simulink model "testControlWithDroneSwarm"  (R2021b)
settings: Solver=ode4  StartTime=0.0  StopTime=inf  FixedStep=sample_time_base  RelTol=1e-3
InitFcn:
  | init_condition();
StopFcn:
  | stop_function();
values from neighbouring files (symbols this model uses):
  flag_alg = params.swarm_algorithm_type    [init_condition.m]
  inertia = inertia'    [init_condition.m]
  kd_att = kd_att'    [init_condition.m]
  kp_att = kp_att'    [init_condition.m]
  lb_pos_pid = lb_pos_pid'    [init_condition.m]
  lb_vel_pid = lb_vel_pid'    [init_condition.m]
  local_ip = '127.0.0.1'    [init_condition.m]
  motor_init_con = states_omeges(14:17,:)    [init_condition.m]
  number = size(position0,2)    [init_condition.m]
  sample_time_base = 0.0025    [init_condition.m]
  sample_time_control = params.sample_time_control_upper    [init_condition.m]
  sim_quad = param_simulink.sim_quad    [init_condition.m]
  target_ip_array = ones(1,number)*1    [init_condition.m]
  ub_pos_pid = ub_pos_pid'    [init_condition.m]
  ub_vel_pid = ub_vel_pid'    [init_condition.m]
  vehicle_int_con = states_omeges(1:13,:)    [init_condition.m]
undefined symbols (not defined in the file or in its folder): a_max_h, a_max_v, cd_filter_pos, cd_filter_vel, cm, ct, euler_max, get_array_slice, gravity, len_arm, map3d_faces, map3d_struct, mass, T_rotor_inverse, thrust_max, v_max_h, v_max_v, yaw_rate_max
libraries: dspindex x8, aerolibanimutils x1
settings Model: Creator=huangjialei  LastModifiedBy=huangjialei

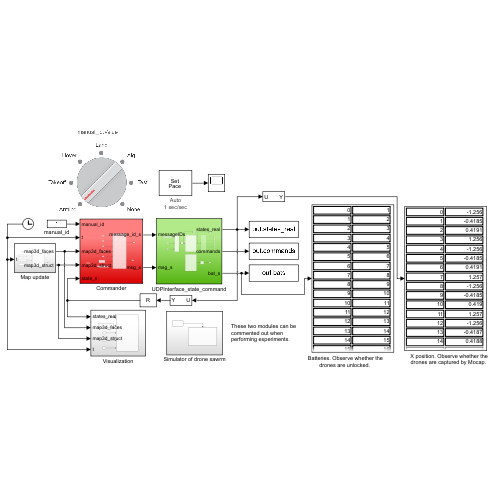
[thumbnail: Simulink's stored preview of the top-level diagram]
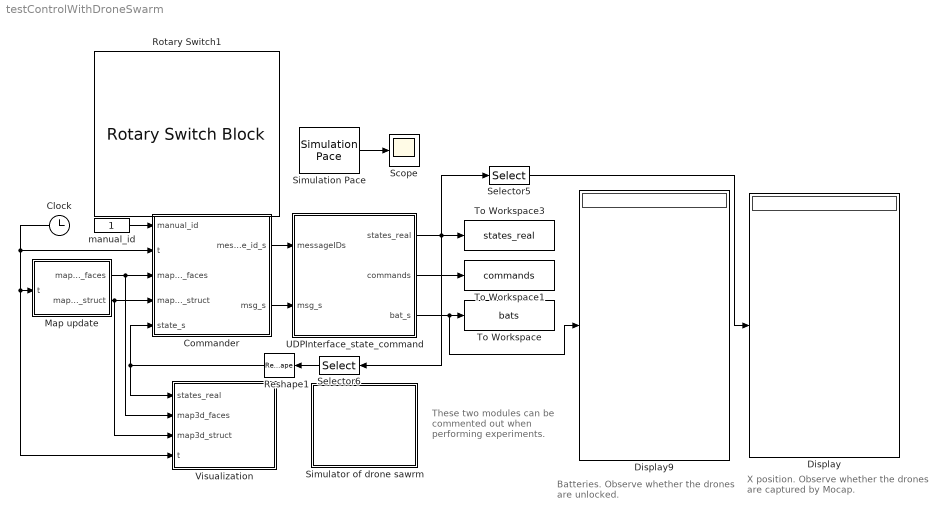
== system testControlWithDroneSwarm ==
  note: These two modules can be commented out when performing experiments.
  note: Batteries. Observe whether the drones are unlocked.
  note: X position. Observe whether the drones are captured by Mocap.
  Clock : Clock
  Commander : Subsystem
  Display : Display
  Display9 : Display
  Map update : Subsystem
  Reshape1 : Reshape  OutputDimensionality=Customize  OutputDimensions=[12,number]
  Rotary Switch1 : RotarySwitchBlock
      settings: Values={{'Arming', 'Takeoff', 'Hover', 'Land', 'Alg', 'Test', 'None'}, [1 2 3 4 5 6 1111]}
  Scope : Scope
  Selector5 : Selector  InputPortWidth=17*number  IndexOptions=Index vector (dialog)  Indices=get_array_slice([1,6], number, 17)  OutputSizes=1
  Selector6 : Selector  InputPortWidth=17*number  IndexOptions=Index vector (dialog)  Indices=get_array_slice(6:17, number, 17)  OutputSizes=1
  Simulation Pace : aerolibanimutils/Simulation Pace  SimulationPace=1  SleepMode=Auto  OutputPaceError=on  SampleTime=sample_time_control
  Simulator of drone sawrm : Subsystem
  To Workspace : ToWorkspace  VariableName=bats  SaveFormat=Timeseries  SampleTime=-1
  To Workspace1 : ToWorkspace  VariableName=commands  SaveFormat=Timeseries  SampleTime=-1
  To Workspace3 : ToWorkspace  VariableName=states_real  SaveFormat=Timeseries  SampleTime=-1
  UDPInterface_state_command : Subsystem
  Visualization : Subsystem
  manual_id : Constant
  wires:
  UDPInterface_state_command/1(states_real) -> Selector6/1, To Workspace3/1, Selector5/1
  Commander/2(msg_s) -> UDPInterface_state_command/2(msg_s)
  UDPInterface_state_command/2(commands) -> To Workspace1/1
  Commander/1(message_id_s) -> UDPInterface_state_command/1(messageIDs)
  UDPInterface_state_command/3(bat_s) -> Display9/1, To Workspace/1
  Selector5/1 -> Display/1
  manual_id/1 -> Commander/1(manual_id)
  Selector6/1 -> Reshape1/1
  Reshape1/1 -> Commander/5(state_s), Visualization/1(states_real)
  Simulation Pace/1 -> Scope/1
  Map update/1(map3d_faces) -> Visualization/2(map3d_faces), Commander/3(map3d_faces)
  Map update/2(map3d_struct) -> Visualization/3(map3d_struct), Commander/4(map3d_struct)
  Clock/1 -> Visualization/4(t), Map update/1(t), Commander/2(t)

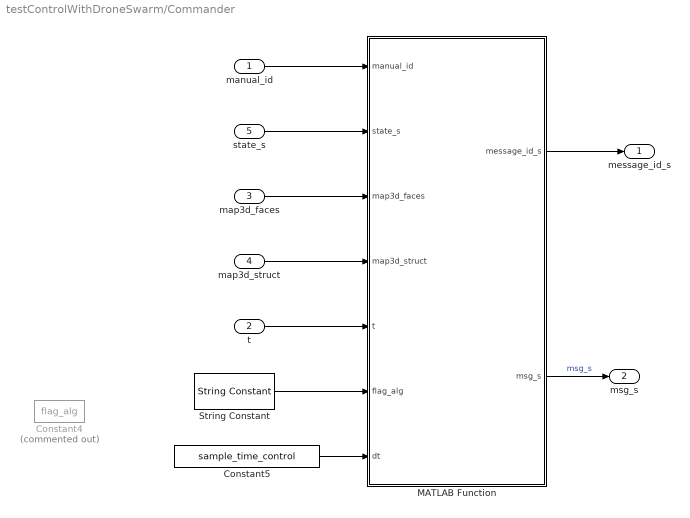
== system testControlWithDroneSwarm/Commander ==
  manual_id : Inport
  t : Inport  Port=2
  map3d_faces : Inport  Port=3
  map3d_struct : Inport  Port=4
  state_s : Inport  Port=5
  Constant4 : Constant  Commented=on  Value=flag_alg
  Constant5 : Constant  Value=sample_time_control
  MATLAB Function : MATLAB Function  TreatAsAtomicUnit=on  SystemSampleTime=sample_time_control
  String Constant : StringConstant  String=flag_alg
  message_id_s : Outport
  msg_s : Outport  Port=2
  wires:
  MATLAB Function/2(msg_s) -> msg_s/1  "msg_s"
  manual_id/1 -> MATLAB Function/1(manual_id)
  t/1 -> MATLAB Function/5(t)
  map3d_faces/1 -> MATLAB Function/3(map3d_faces)
  map3d_struct/1 -> MATLAB Function/4(map3d_struct)
  MATLAB Function/1(message_id_s) -> message_id_s/1
  String Constant/1 -> MATLAB Function/6(flag_alg)
  Constant5/1 -> MATLAB Function/7(dt)
  state_s/1 -> MATLAB Function/2(state_s)

== system testControlWithDroneSwarm/Map update ==
  t : Inport
  Constant : Constant  Value=sample_time_control
  Constant1 : Constant  Value=map3d_faces
  Constant2 : Constant  Value=map3d_struct
  MATLAB Function : MATLAB Function  TreatAsAtomicUnit=on  SystemSampleTime=sample_time_control
  map3d_faces : Outport
  map3d_struct : Outport  Port=2
  wires:
  MATLAB Function/1(map3d_faces) -> map3d_faces/1
  MATLAB Function/2(map3d_struct) -> map3d_struct/1
  t/1 -> MATLAB Function/1(t)
  Constant/1 -> MATLAB Function/2(sample_time_control)
  Constant1/1 -> MATLAB Function/3(map3d_faces_0)
  Constant2/1 -> MATLAB Function/4(map3d_struct_0)

== system testControlWithDroneSwarm/Simulator of drone sawrm ==
  Constant : Constant  Value=sim_quad
  Subsystem : Subsystem
  wires:
  Constant/1 -> Subsystem/Enable

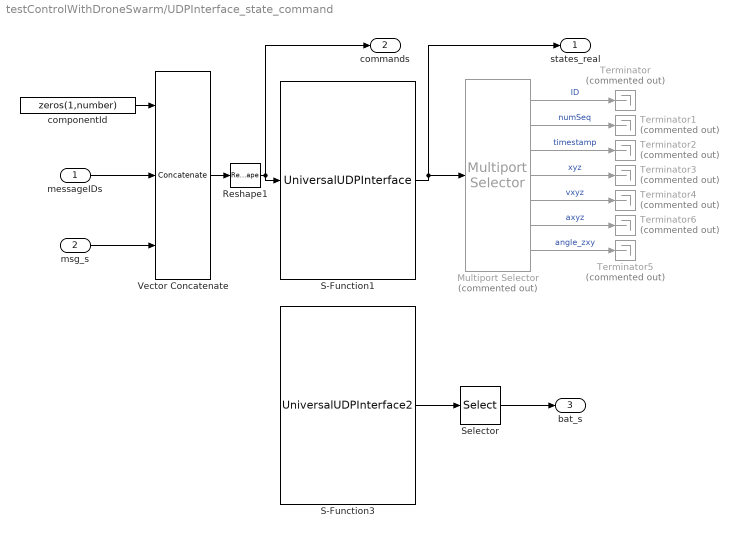
== system testControlWithDroneSwarm/UDPInterface_state_command ==
  messageIDs : Inport
  msg_s : Inport  Port=2
  Multiport Selector : dspindex/Multiport Selector  Commented=on  rowsOrCols=Rows  idxCellArray={1:15:15*number,2:15:15*number,3:15:15*number,repmat(4:6,1,number) + reshape(repmat((0:number-1)*15,3,1),1,3*number), repmat(7:9,1,number) + reshape(repmat((0:number-1)*15,3,1),1,3*number), repmat(10:12,1,number) + reshape(repmat((0:number-1)*15,3,1),1,3*number), repmat(13:15,1,number) + reshape(repmat((0:number-1)*15,3,1),1,3*number)}  idxErrMode=Clip Index
  Reshape1 : Reshape
  S-Function1 : S-Function  FunctionName=UniversalUDPInterface  Parameters=sampleTime,number,portTarget,portLocal,ipTarget,ipLocal,flagSend,flagRecv,inputPortWidth,outputPortWidth  SFunctionDeploymentMode=off  EnableBusSupport=off  mask{number=number, ipLocal=local_ip, ipTarget=target_ip_array, portTarget=21000, portLocal=21000, flagSend=on, flagRecv=on, inputPortWidth=6, outputPortWidth=17, sampleTime=sample_time_control}
      mask prompts: number "Number of vehicles"; ipLocal "Local ip"; ipTarget "Target ip"; portTarget "Start port of target"; portLocal "Start port of local"; flagSend "Enable sender"; flagRecv "Enable receiver"; inputPortWidth "Width of input port"; outputPortWidth "Width of output port"; sampleTime "Sample time"
      mask help:
      | input port: componentId, messageId, msgData[0], msgData[1], ...
      | output port: systemId, numSequence, timeStamp,msgData[0], msgData[1], ...
  S-Function3 : S-Function  FunctionName=UniversalUDPInterface2  Parameters=sampleTime,number,portTarget,portLocal,ipTarget,ipLocal,flagSend,flagRecv,inputPortWidth,outputPortWidth  SFunctionDeploymentMode=off  EnableBusSupport=off  mask{number=number, ipLocal=local_ip, ipTarget=target_ip_array, portTarget=22000, portLocal=20000, flagSend=off, flagRecv=on, inputPortWidth=3, outputPortWidth=6, sampleTime=sample_time_control}
      mask prompts: number "Number of vehicles"; ipLocal "Local ip"; ipTarget "Target ip"; portTarget "Start port of target"; portLocal "Start port of local"; flagSend "Enable sender"; flagRecv "Enable receiver"; inputPortWidth "Width of input port"; outputPortWidth "Width of output port"; sampleTime "Sample time"
      mask help:
      | input port: componentId, messageId, msgData[0], msgData[1], ...
      | output port: systemId, numSequence, timeStamp,msgData[0], msgData[1], ...
  Selector : Selector  InputPortWidth=6*number  IndexOptions=Index vector (dialog)  Indices=get_array_slice([1,6], number, 6)  OutputSizes=1
  Terminator{,1..6} (7 alike) : Terminator  Commented=on
  Vector Concatenate : Concatenate  NumInputs=3  Mode=Multidimensional array
  componentId : Constant  Value=zeros(1,number)  VectorParams1D=off
  states_real : Outport
  commands : Outport  Port=2
  bat_s : Outport  Port=3
  wires:
  Multiport Selector/2 -> Terminator1/1  "numSeq"
  Multiport Selector/5 -> Terminator4/1  "vxyz"
  Vector Concatenate/1 -> Reshape1/1
  Multiport Selector/3 -> Terminator2/1  "timestamp"
  messageIDs/1 -> Vector Concatenate/2
  Reshape1/1 -> S-Function1/1, commands/1
  componentId/1 -> Vector Concatenate/1
  Multiport Selector/4 -> Terminator3/1  "xyz"
  Multiport Selector/1 -> Terminator/1  "ID"
  msg_s/1 -> Vector Concatenate/3
  S-Function3/1 -> Selector/1
  Selector/1 -> bat_s/1
  Multiport Selector/7 -> Terminator5/1  "angle_zxy"
  Multiport Selector/6 -> Terminator6/1  "axyz"
  S-Function1/1 -> states_real/1, Multiport Selector/1

== system testControlWithDroneSwarm/Visualization ==
  states_real : Inport
  map3d_faces : Inport  Port=2
  map3d_struct : Inport  Port=3
  t : Inport  Port=4
  Constant : Constant  Value=sample_time_base
  MATLAB Function : MATLAB Function  TreatAsAtomicUnit=on  SystemSampleTime=sample_time_base
  wires:
  map3d_faces/1 -> MATLAB Function/4(map3d_faces)
  map3d_struct/1 -> MATLAB Function/5(map3d_struct)
  states_real/1 -> MATLAB Function/3(states)
  t/1 -> MATLAB Function/1(t)
  Constant/1 -> MATLAB Function/2(dt)

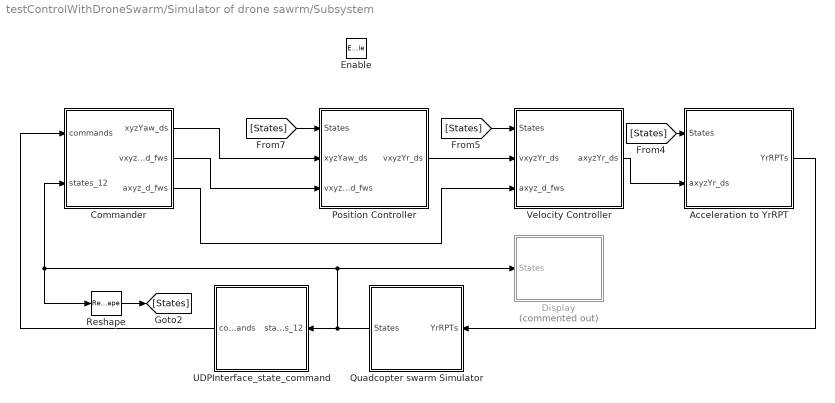
== system testControlWithDroneSwarm/Simulator of drone sawrm/Subsystem ==
  Enable : EnablePort
  Acceleration to YrRPT : Subsystem
  Commander : Subsystem
  Display : Subsystem  Commented=on
  Position Controller : Subsystem
  Quadcopter swarm Simulator : Subsystem
  Reshape : Reshape
  UDPInterface_state_command : Subsystem
  Velocity Controller : Subsystem
  wires:
  Velocity Controller/1(axyzYr_ds) -> Acceleration to YrRPT/2(axyzYr_ds)
  Quadcopter swarm Simulator/1(States) -> UDPInterface_state_command/1(states_12), Commander/2(states_12), Reshape/1, Display/1(States)
  Commander/1(xyzYaw_ds) -> Position Controller/2(xyzYaw_ds)
  Position Controller/1(vxyzYr_ds) -> Velocity Controller/2(vxyzYr_ds)
  UDPInterface_state_command/1(commands) -> Commander/1(commands)
  Reshape/1 -> [States]
  [States] -> Velocity Controller/1(States)
  [States] -> Acceleration to YrRPT/1(States)
  Commander/2(vxyzYr_d_fws) -> Position Controller/3(vxyzYr_d_fws)
  [States] -> Position Controller/1(States)
  Acceleration to YrRPT/1(YrRPTs) -> Quadcopter swarm Simulator/1(YrRPTs)
  Commander/3(axyz_d_fws) -> Velocity Controller/3(axyz_d_fws)

== system testControlWithDroneSwarm/Simulator of drone sawrm/Subsystem/Acceleration to YrRPT ==
  States : Inport
  axyzYr_ds : Inport  Port=2
  Selector : Selector  InputPortWidth=12*number  IndexOptions=Index vector (dialog)  Indices=10:12:12*number  OutputSizes=1
  Subsystem12 : Subsystem
  YrRPTs : Outport
  wires:
  States/1 -> Selector/1
  Selector/1 -> Subsystem12/2(yaws)
  Subsystem12/1(YrRPT) -> YrRPTs/1  "YrRPT"
  axyzYr_ds/1 -> Subsystem12/1(axyzYr_ds)

== system testControlWithDroneSwarm/Simulator of drone sawrm/Subsystem/Commander ==
  commands : Inport
  states_12 : Inport  Port=2
  Clock : Clock
  MATLAB Function : MATLAB Function  TreatAsAtomicUnit=on  SystemSampleTime=sample_time_control
  xyzYaw_ds : Outport
  vxyzYr_d_fws : Outport  Port=2
  axyz_d_fws : Outport  Port=3
  wires:
  Clock/1 -> MATLAB Function/3(t)
  MATLAB Function/2(vxyzYr_ds_fw) -> vxyzYr_d_fws/1
  MATLAB Function/1(xyzYaw_ds) -> xyzYaw_ds/1
  MATLAB Function/3(axyz_ds_fw) -> axyz_d_fws/1
  states_12/1 -> MATLAB Function/2(states)
  commands/1 -> MATLAB Function/1(commands)

== system testControlWithDroneSwarm/Simulator of drone sawrm/Subsystem/Display ==
  States : Inport
  Clock : Clock
  Constant : Constant  Value=len_arm
  MATLAB Function : MATLAB Function  TreatAsAtomicUnit=on  SystemSampleTime=0.1
  wires:
  Constant/1 -> MATLAB Function/2(lenArm)
  Clock/1 -> MATLAB Function/3(t)
  States/1 -> MATLAB Function/1(states)

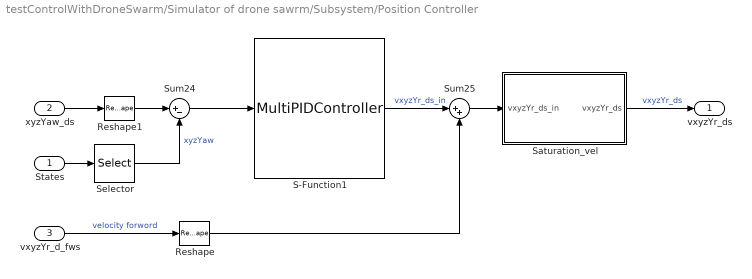
== system testControlWithDroneSwarm/Simulator of drone sawrm/Subsystem/Position Controller ==
  States : Inport
  xyzYaw_ds : Inport  Port=2
  vxyzYr_d_fws : Inport  Port=3
  Reshape : Reshape
  Reshape1 : Reshape
  S-Function1 : S-Function  FunctionName=MultiPIDController  Parameters=sampleTime,number,width,enable_P,enable_I,enable_D,proportion,integral,derivative,c,enable_reset,lb,ub  SFunctionDeploymentMode=off  EnableBusSupport=off  mask{number=number, width=4, enable_P=on, enable_I=on, enable_D=on, proportion=[1,1,1,0], integral=[0,0,0,0], derivative=[0,0,3,0], c=cd_filter_pos, enable_reset=off, lb=lb_pos_pid, ub=ub_pos_pid, sampleTime=sample_time_base}
      mask prompts: number "Number of input port"; width "Width of per input"; enable_P "Enable P"; enable_I "Enable I"; enable_D "Enable D"; c "Coefficient of low-pass filter in derivative part"; enable_reset "Rising edge reset of integral"; lb "Lower boundary of outputs"; ub "Upper boundary of outputs"; sampleTime "Sample time"
      mask Callback enable_P:
      | % disp(get_param(gcbh,'enable_P'))
      | % if strcmp(get_param(gcbh,'enable_P'), 'off')
      | %    disp(get_param(gcbh,'ParameterGroupVar'))
      | %
      | % end
  Saturation_vel : Subsystem
  Selector : Selector  InputPortWidth=12*number  IndexOptions=Index vector (dialog)  Indices=repmat([1,2,3,10],1,number) + reshape(repmat((0:number-1)*12,4,1),1,4*number)  OutputSizes=1
  Sum24 : Sum  Inputs=|+-
  Sum25 : Sum  Inputs=|++
  vxyzYr_ds : Outport
  wires:
  xyzYaw_ds/1 -> Reshape1/1
  States/1 -> Selector/1
  vxyzYr_d_fws/1 -> Reshape/1  "velocity forword"
  Sum24/1 -> S-Function1/1
  Selector/1 -> Sum24/2  "xyzYaw"
  S-Function1/1 -> Sum25/1  "vxyzYr_ds_in"
  Sum25/1 -> Saturation_vel/1(vxyzYr_ds_in)
  Saturation_vel/1(vxyzYr_ds) -> vxyzYr_ds/1  "vxyzYr_ds"
  Reshape/1 -> Sum25/2
  Reshape1/1 -> Sum24/1

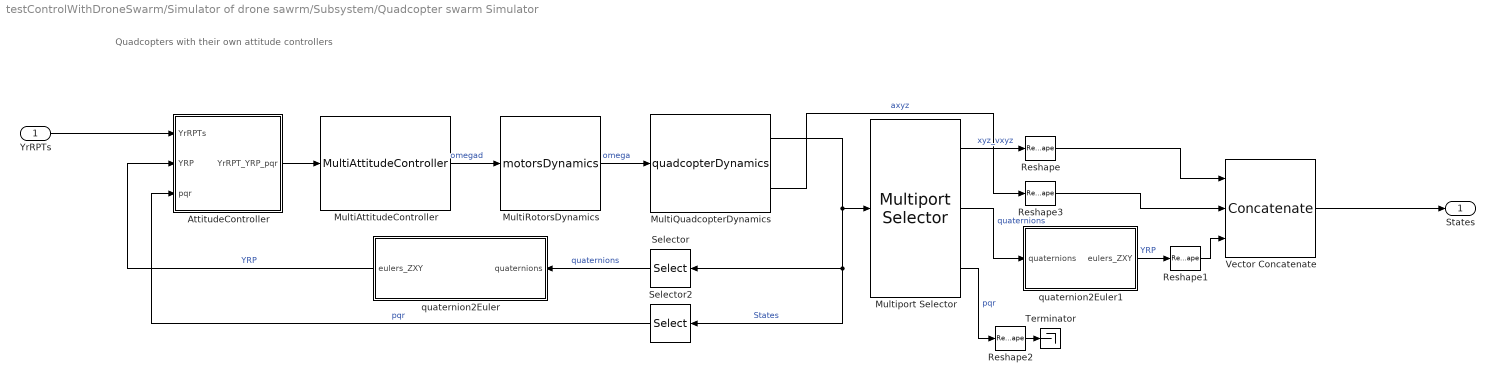
== system testControlWithDroneSwarm/Simulator of drone sawrm/Subsystem/Quadcopter swarm Simulator ==
  note: Quadcopters with their own attitude controllers
  YrRPTs : Inport
  AttitudeController : Subsystem
  MultiAttitudeController : S-Function  FunctionName=MultiAttitudeController  Parameters=number_a,I_a,kp_a,kd_a,arm_length_a,ct_a,cm_a  SFunctionDeploymentMode=off  EnableBusSupport=off  mask{number_a=number+0, I_a=inertia, kp_a=kp_att, kd_a=kd_att, arm_length_a=len_arm, ct_a=ct, cm_a=cm}
      mask prompts: number_a "Number of quadcopters"; I_a "Moment of inertia"; kp_a "Coefficient of proportions"; kd_a "Coefficient of derivatives"; arm_length_a "Length of arm"; ct_a "Thrust coefficient of propeller"; cm_a "Moment coefficient of propeller"
      mask Display:
      | % number = get_param(gcbh,'number_a');
      | % for i = 1:str2num(number)
      | %    port_label('input', i, ['YrRPT_YRP_pqr',num2str(i)]);
      | % end
      | % for i = 1:str2num(number)
      | %    port_label('output', i, ['RPM_d',num2str(i)]);
      | % end
  MultiQuadcopterDynamics : S-Function  FunctionName=quadcopterDynamics  Parameters=number_q,mass_q,I_q,arm_length_q,ct_q,cm_q,conInit_q  SFunctionDeploymentMode=off  EnableBusSupport=off  mask{number_q=number+0, mass_q=mass, I_q=inertia, arm_length_q=len_arm, ct_q=ct, cm_q=cm, conInit_q=vehicle_int_con}
      mask prompts: number_q "Number of quadcopters"; mass_q "Mass"; I_q "Moment of inertia"; arm_length_q "Length of arm"; ct_q "Thrust coefficient of propeller"; cm_q "Moment coefficient of propeller"; conInit_q "Initial condition"
      mask Display:
      | number = get_param(gcbh,'number_q');
      | for i = 1:str2num(number)
      |    port_label('output', i, ['State',num2str(i)]);
      | end
      | for i = 1:str2num(number)
      |    port_label('input', i, ['RPM',num2str(i)]);
      | end
  MultiRotorsDynamics : S-Function  FunctionName=motorsDynamics  Parameters=number_m,K_m,conInit_m  SFunctionDeploymentMode=off  EnableBusSupport=off  mask{number_m=number+0, K_m=T_rotor_inverse, conInit_m=motor_init_con}
      mask prompts: number_m "Number of quadcopters"; K_m "Reciprocal of time constant"; conInit_m "Initial condition"
      mask Display:
      | number = get_param(gcbh,'number_m');
      | for i = 1:str2num(number)
      |    port_label('output', i, ['RPM',num2str(i)]);
      | end
      | for i = 1:str2num(number)
      |    port_label('input', i, ['RPM_d',num2str(i)]);
      | end
  Multiport Selector : dspindex/Multiport Selector  rowsOrCols=Rows  idxCellArray={ repmat(1:6,1,number) + reshape(repmat((0:number-1)*13,6,1),1,6*number),repmat(7:10,1,number) + reshape(repmat((0:number-1)*13,4,1),1,4*number), repmat(11:13,1,number) + reshape(repmat((0:number-1)*13,3,1),1,3*number)}  idxErrMode=Clip Index
  Reshape : Reshape  OutputDimensionality=Customize  OutputDimensions=[6,number]
  Reshape1 : Reshape  OutputDimensionality=Customize  OutputDimensions=[3,number]
  Reshape2 : Reshape  OutputDimensionality=Customize  OutputDimensions=[3,number]
  Reshape3 : Reshape  OutputDimensionality=Customize  OutputDimensions=[3,number]
  Selector : Selector  InputPortWidth=13*number  IndexOptions=Index vector (dialog)  Indices=repmat([7,8,9,10],1,number) + reshape(repmat((0:number-1)*13,4,1),1,4*number)  OutputSizes=1
  Selector2 : Selector  InputPortWidth=13*number  IndexOptions=Index vector (dialog)  Indices=repmat([11,12,13],1,number) + reshape(repmat((0:number-1)*13,3,1),1,3*number)  OutputSizes=1
  Terminator : Terminator
  Vector Concatenate : Concatenate  NumInputs=3  Mode=Multidimensional array
  quaternion2Euler : Subsystem
  quaternion2Euler1 : Subsystem
  States : Outport
  wires:
  YrRPTs/1 -> AttitudeController/1(YrRPTs)
  Selector/1 -> quaternion2Euler/1(quaternions)  "quaternions"
  quaternion2Euler/1(eulers_ZXY) -> AttitudeController/2(YRP)  "YRP"
  Selector2/1 -> AttitudeController/3(pqr)  "pqr"
  MultiAttitudeController/1 -> MultiRotorsDynamics/1  "omegad"
  MultiRotorsDynamics/1 -> MultiQuadcopterDynamics/1  "omega"
  MultiQuadcopterDynamics/1 -> Multiport Selector/1, Selector2/1, Selector/1  "States"
  Multiport Selector/2 -> quaternion2Euler1/1(quaternions)  "quaternions"
  Multiport Selector/1 -> Reshape/1  "xyz_vxyz"
  Reshape/1 -> Vector Concatenate/1
  quaternion2Euler1/1(eulers_ZXY) -> Reshape1/1  "YRP"
  Multiport Selector/3 -> Reshape2/1  "pqr"
  AttitudeController/1(YrRPT_YRP_pqr) -> MultiAttitudeController/1
  Vector Concatenate/1 -> States/1
  Reshape2/1 -> Terminator/1
  Reshape1/1 -> Vector Concatenate/3
  MultiQuadcopterDynamics/2 -> Reshape3/1  "axyz"
  Reshape3/1 -> Vector Concatenate/2

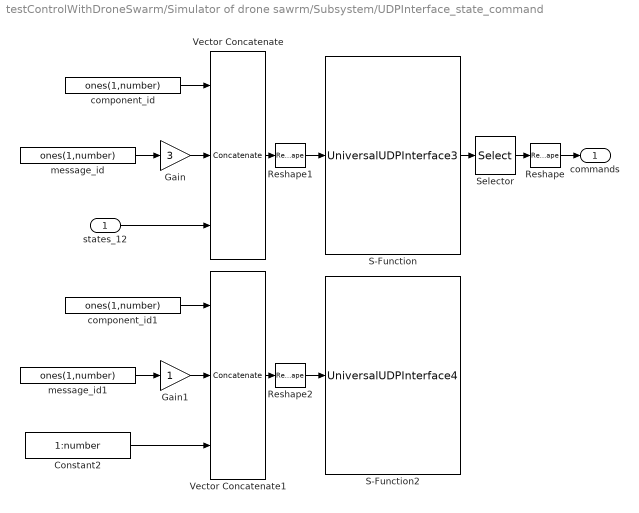
== system testControlWithDroneSwarm/Simulator of drone sawrm/Subsystem/UDPInterface_state_command ==
  states_12 : Inport
  Constant2 : Constant  Value=1:number  VectorParams1D=off
  Gain : Gain  Gain=3
  Gain1 : Gain
  Reshape : Reshape  OutputDimensionality=Customize  OutputDimensions=[6,number]
  Reshape1 : Reshape
  Reshape2 : Reshape
  S-Function : S-Function  FunctionName=UniversalUDPInterface3  Parameters=sampleTime,number,portTarget,portLocal,ipTarget,ipLocal,flagSend,flagRecv,inputPortWidth,outputPortWidth  SFunctionDeploymentMode=off  EnableBusSupport=off  mask{number=number, ipLocal=local_ip, ipTarget=target_ip_array, portTarget=20999, portLocal=21001, flagSend=on, flagRecv=on, inputPortWidth=14, outputPortWidth=9, sampleTime=sample_time_control}
      mask prompts: number "Number of vehicles"; ipLocal "Local ip"; ipTarget "Target ip"; portTarget "Start port of target"; portLocal "Start port of local"; flagSend "Enable sender"; flagRecv "Enable receiver"; inputPortWidth "Width of input port"; outputPortWidth "Width of output port"; sampleTime "Sample time"
      mask help:
      | input port: componentId, messageId, msgData[0], msgData[1], ...
      | output port: systemId, numSequence, timeStamp,msgData[0], msgData[1], ...
  S-Function2 : S-Function  FunctionName=UniversalUDPInterface4  Parameters=sampleTime,number,portTarget,portLocal,ipTarget,ipLocal,flagSend,flagRecv,inputPortWidth,outputPortWidth  SFunctionDeploymentMode=off  EnableBusSupport=off  mask{number=number, ipLocal=local_ip, ipTarget=target_ip_array, portTarget=19999, portLocal=22001, flagSend=on, flagRecv=off, inputPortWidth=3, outputPortWidth=9, sampleTime=sample_time_control}
      mask prompts: number "Number of vehicles"; ipLocal "Local ip"; ipTarget "Target ip"; portTarget "Start port of target"; portLocal "Start port of local"; flagSend "Enable sender"; flagRecv "Enable receiver"; inputPortWidth "Width of input port"; outputPortWidth "Width of output port"; sampleTime "Sample time"
      mask help:
      | input port: componentId, messageId, msgData[0], msgData[1], ...
      | output port: systemId, numSequence, timeStamp,msgData[0], msgData[1], ...
  Selector : Selector  InputPortWidth=9*number  IndexOptions=Index vector (dialog)  Indices=get_array_slice(4:9, number, 9)  OutputSizes=1
  Vector Concatenate : Concatenate  NumInputs=3  Mode=Multidimensional array
  Vector Concatenate1 : Concatenate  NumInputs=3  Mode=Multidimensional array
  component_id : Constant  Value=ones(1,number)  VectorParams1D=off
  component_id1 : Constant  Value=ones(1,number)  VectorParams1D=off
  message_id : Constant  Value=ones(1,number)  VectorParams1D=off
  message_id1 : Constant  Value=ones(1,number)  VectorParams1D=off
  commands : Outport
  wires:
  Vector Concatenate/1 -> Reshape1/1
  Reshape1/1 -> S-Function/1
  component_id/1 -> Vector Concatenate/1
  message_id/1 -> Gain/1
  Gain/1 -> Vector Concatenate/2
  S-Function/1 -> Selector/1
  Gain1/1 -> Vector Concatenate1/2
  message_id1/1 -> Gain1/1
  Constant2/1 -> Vector Concatenate1/3
  component_id1/1 -> Vector Concatenate1/1
  Reshape2/1 -> S-Function2/1
  Vector Concatenate1/1 -> Reshape2/1
  states_12/1 -> Vector Concatenate/3
  Selector/1 -> Reshape/1
  Reshape/1 -> commands/1

== system testControlWithDroneSwarm/Simulator of drone sawrm/Subsystem/Velocity Controller ==
  States : Inport
  vxyzYr_ds : Inport  Port=2
  axyz_d_fws : Inport  Port=3
  Multiport Selector : dspindex/Multiport Selector  rowsOrCols=Rows  idxCellArray={ repmat([1,2,3],1,number) + reshape(repmat((0:number-1)*4,3,1),1,3*number),4:4:4*number}  idxErrMode=Clip Index
  Reshape : Reshape
  S-Function2 : S-Function  FunctionName=MultiPIDController  Parameters=sampleTime,number,width,enable_P,enable_I,enable_D,proportion,integral,derivative,c,enable_reset,lb,ub  SFunctionDeploymentMode=off  EnableBusSupport=off  mask{number=number+0, width=3, enable_P=on, enable_I=on, enable_D=on, proportion=[1.2,1.2,1], integral=[2,2,0.8], derivative=[0.3,0.3,0], c=cd_filter_vel, enable_reset=off, lb=lb_vel_pid, ub=ub_vel_pid, sampleTime=sample_time_base}
      mask prompts: number "Number of input port"; width "Width of per input"; enable_P "Enable P"; enable_I "Enable I"; enable_D "Enable D"; c "Coefficient of low-pass filter in derivative part"; enable_reset "Rising edge reset of integral"; lb "Lower boundary of outputs"; ub "Upper boundary of outputs"; sampleTime "Sample time"
      mask Callback enable_P:
      | % disp(get_param(gcbh,'enable_P'))
      | % if strcmp(get_param(gcbh,'enable_P'), 'off')
      | %    disp(get_param(gcbh,'ParameterGroupVar'))
      | %
      | % end
  Saturation_Acc : Subsystem
  Selector : Selector  InputPortWidth=12*number  IndexOptions=Index vector (dialog)  Indices=repmat([4,5,6],1,number) + reshape(repmat((0:number-1)*12,3,1),1,3*number)  OutputSizes=1
  Sum1 : Sum  Inputs=|++
  Sum2 : Sum  Inputs=|+-
  axyzYr_ds : Outport
  wires:
  States/1 -> Selector/1
  Selector/1 -> Sum2/2  "vxyz"
  Sum2/1 -> S-Function2/1
  Multiport Selector/1 -> Sum2/1  "vxyz_d"
  Multiport Selector/2 -> Saturation_Acc/2(yaw_rates)  "yaw_rate_d"
  vxyzYr_ds/1 -> Multiport Selector/1
  Saturation_Acc/1(axyzYr_ds) -> axyzYr_ds/1  "axyzYs_ds"
  S-Function2/1 -> Sum1/1  "axyzYr_ds_in"
  Sum1/1 -> Saturation_Acc/1(axyz_d_in)
  axyz_d_fws/1 -> Reshape/1
  Reshape/1 -> Sum1/2

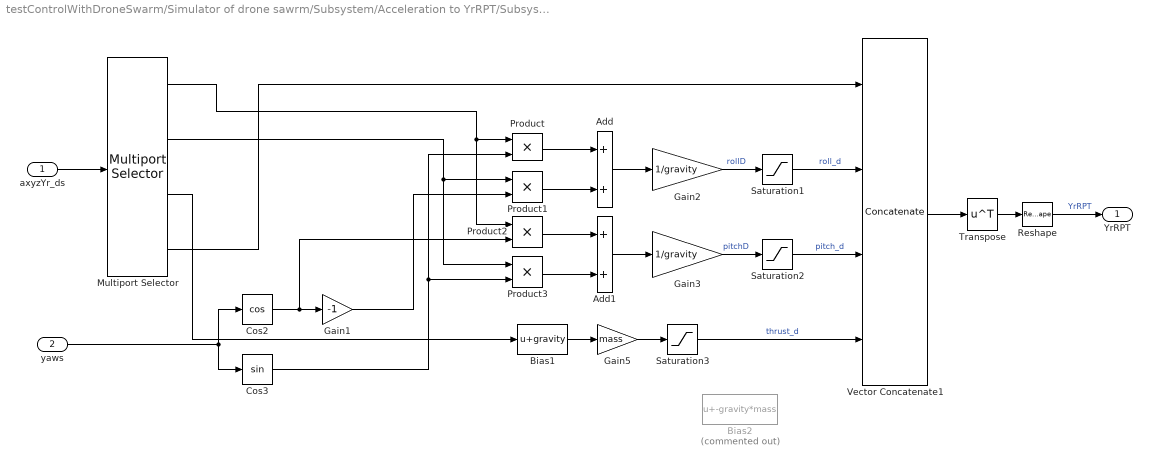
== system testControlWithDroneSwarm/Simulator of drone sawrm/Subsystem/Acceleration to YrRPT/Subsystem12 ==
  axyzYr_ds : Inport
  yaws : Inport  Port=2
  Add : Sum
  Add1 : Sum
  Bias1 : Bias  Bias=gravity
  Bias2 : Bias  Commented=on  Bias=-gravity*mass
  Cos2 : Trigonometry  Operator=cos
  Cos3 : Trigonometry
  Gain1 : Gain  Gain=-1
  Gain2 : Gain  Gain=1/gravity
  Gain3 : Gain  Gain=1/gravity
  Gain5 : Gain  Gain=mass
  Multiport Selector : dspindex/Multiport Selector  rowsOrCols=Rows  idxCellArray={ 1:4:4*number,2:4:4*number, 3:4:4*number,4:4:4*number}  idxErrMode=Clip Index
  Product{,1..3} (4 alike) : Product
  Reshape : Reshape
  Saturation1 : Saturate  UpperLimit=euler_max  LowerLimit=-euler_max
  Saturation2 : Saturate  UpperLimit=euler_max  LowerLimit=-euler_max
  Saturation3 : Saturate  UpperLimit=thrust_max  LowerLimit=0
  Transpose : Math  Operator=transpose  SaturateOnIntegerOverflow=on
  Vector Concatenate1 : Concatenate  NumInputs=4  Mode=Multidimensional array  ConcatenateDimension=2
  YrRPT : Outport
  wires:
  Saturation3/1 -> Vector Concatenate1/4  "thrust_d"
  Saturation2/1 -> Vector Concatenate1/3  "pitch_d"
  Saturation1/1 -> Vector Concatenate1/2  "roll_d"
  Gain5/1 -> Saturation3/1
  Multiport Selector/4 -> Vector Concatenate1/1
  Reshape/1 -> YrRPT/1  "YrRPT"
  Gain2/1 -> Saturation1/1  "rollD"
  Add/1 -> Gain2/1
  Multiport Selector/1 -> Product/1, Product2/1
  Gain1/1 -> Product1/2
  Product/1 -> Add/1
  axyzYr_ds/1 -> Multiport Selector/1
  Product3/1 -> Add1/2
  Cos2/1 -> Gain1/1, Product2/2
  Product1/1 -> Add/2
  Multiport Selector/3 -> Bias1/1
  Gain3/1 -> Saturation2/1  "pitchD"
  Product2/1 -> Add1/1
  Multiport Selector/2 -> Product1/1, Product3/1
  Cos3/1 -> Product3/2, Product/2
  Add1/1 -> Gain3/1
  yaws/1 -> Cos2/1, Cos3/1
  Bias1/1 -> Gain5/1
  Vector Concatenate1/1 -> Transpose/1
  Transpose/1 -> Reshape/1

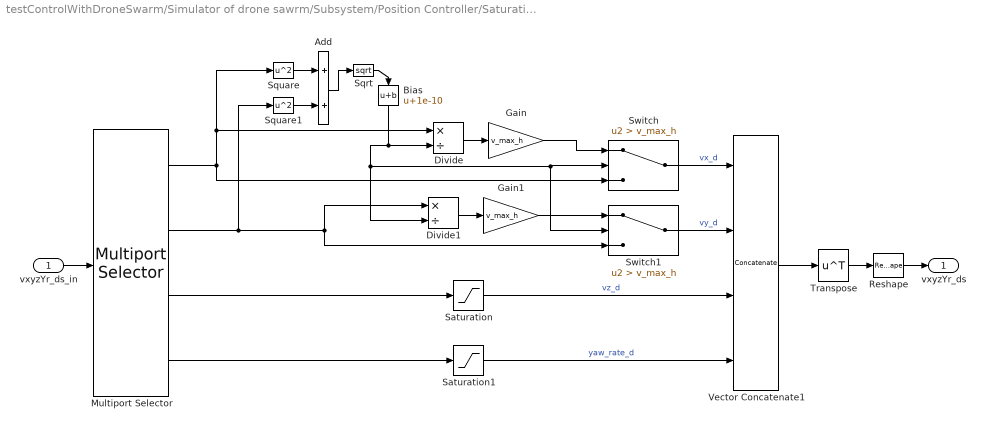
== system testControlWithDroneSwarm/Simulator of drone sawrm/Subsystem/Position Controller/Saturation_vel ==
  vxyzYr_ds_in : Inport
  Add : Sum
  Bias : Bias  Bias=1e-10
  Divide : Product  Inputs=*/
  Divide1 : Product  Inputs=*/
  Gain : Gain  Gain=v_max_h
  Gain1 : Gain  Gain=v_max_h
  Multiport Selector : dspindex/Multiport Selector  rowsOrCols=Rows  idxCellArray={ 1:4:4*number,2:4:4*number, 3:4:4*number, 4:4:4*number }  idxErrMode=Clip Index
  Reshape : Reshape
  Saturation : Saturate  UpperLimit=v_max_v  LowerLimit=-v_max_v
  Saturation1 : Saturate  UpperLimit=yaw_rate_max  LowerLimit=-yaw_rate_max
  Sqrt : Sqrt  SaturateOnIntegerOverflow=on
  Square : Math  Operator=square  SaturateOnIntegerOverflow=on
  Square1 : Math  Operator=square  SaturateOnIntegerOverflow=on
  Switch : Switch  Criteria=u2 > Threshold  Threshold=v_max_h
  Switch1 : Switch  Criteria=u2 > Threshold  Threshold=v_max_h
  Transpose : Math  Operator=transpose  SaturateOnIntegerOverflow=on
  Vector Concatenate1 : Concatenate  NumInputs=4  Mode=Multidimensional array  ConcatenateDimension=2
  vxyzYr_ds : Outport
  wires:
  Switch/1 -> Vector Concatenate1/1  "vx_d"
  Multiport Selector/3 -> Saturation/1
  Gain/1 -> Switch/1
  Divide/1 -> Gain/1
  Multiport Selector/1 -> Square/1, Divide/1, Switch/3
  Add/1 -> Sqrt/1
  Square1/1 -> Add/2
  Square/1 -> Add/1
  vxyzYr_ds_in/1 -> Multiport Selector/1
  Multiport Selector/4 -> Saturation1/1
  Saturation1/1 -> Vector Concatenate1/4  "yaw_rate_d"
  Saturation/1 -> Vector Concatenate1/3  "vz_d"
  Sqrt/1 -> Bias/1
  Multiport Selector/2 -> Divide1/1, Switch1/3, Square1/1
  Divide1/1 -> Gain1/1
  Gain1/1 -> Switch1/1
  Switch1/1 -> Vector Concatenate1/2  "vy_d"
  Vector Concatenate1/1 -> Transpose/1
  Transpose/1 -> Reshape/1
  Reshape/1 -> vxyzYr_ds/1
  Bias/1 -> Divide/2, Divide1/2, Switch/2, Switch1/2

== system testControlWithDroneSwarm/Simulator of drone sawrm/Subsystem/Quadcopter swarm Simulator/AttitudeController ==
  YrRPTs : Inport
  YRP : Inport  Port=2
  pqr : Inport  Port=3
  Reshape : Reshape  OutputDimensionality=Customize  OutputDimensions=[4,number]
  Reshape1 : Reshape  OutputDimensionality=Customize  OutputDimensions=[3,number]
  Reshape2 : Reshape  OutputDimensionality=Customize  OutputDimensions=[3,number]
  Reshape3 : Reshape
  Vector Concatenate : Concatenate  NumInputs=3  Mode=Multidimensional array
  YrRPT_YRP_pqr : Outport
  wires:
  YrRPTs/1 -> Reshape/1
  YRP/1 -> Reshape1/1
  pqr/1 -> Reshape2/1
  Reshape/1 -> Vector Concatenate/1
  Reshape1/1 -> Vector Concatenate/2
  Reshape2/1 -> Vector Concatenate/3
  Vector Concatenate/1 -> Reshape3/1
  Reshape3/1 -> YrRPT_YRP_pqr/1

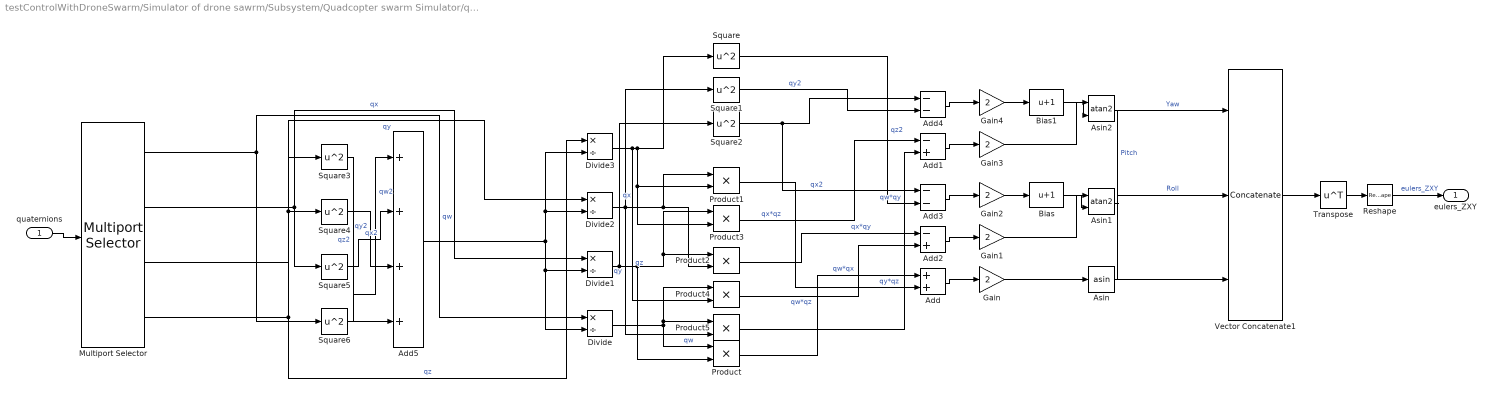
== system testControlWithDroneSwarm/Simulator of drone sawrm/Subsystem/Quadcopter swarm Simulator/quaternion2Euler ==
  quaternions : Inport
  Add : Sum
  Add1 : Sum  Inputs=-+
  Add2 : Sum  Inputs=-+
  Add3 : Sum  Inputs=--
  Add4 : Sum  Inputs=--
  Add5 : Sum  Inputs=++++
  Asin : Trigonometry  Operator=asin
  Asin1 : Trigonometry  Operator=atan2
  Asin2 : Trigonometry  Operator=atan2
  Bias : Bias  Bias=1
  Bias1 : Bias  Bias=1
  Divide{,1..3} (4 alike) : Product  Inputs=*/
  Gain{,1..4} (5 alike) : Gain  Gain=2
  Multiport Selector : dspindex/Multiport Selector  rowsOrCols=Rows  idxCellArray={ 1:4:4*number,2:4:4*number, 3:4:4*number, 4:4:4*number }  idxErrMode=Clip Index
  Product{,1..5} (6 alike) : Product
  Reshape : Reshape
  Square{,1..6} (7 alike) : Math  Operator=square  SaturateOnIntegerOverflow=on
  Transpose : Math  Operator=transpose  SaturateOnIntegerOverflow=on
  Vector Concatenate1 : Concatenate  NumInputs=3  Mode=Multidimensional array  ConcatenateDimension=2
  eulers_ZXY : Outport
  wires:
  Multiport Selector/1 -> Divide/1, Square6/1  "qw"
  Add5/1 -> Divide1/2, Divide/2, Divide3/2, Divide2/2
  Square4/1 -> Add5/3  "qy2"
  Add/1 -> Gain/1
  quaternions/1 -> Multiport Selector/1
  Multiport Selector/4 -> Divide3/1, Square3/1  "qz"
  Product/1 -> Add/1  "qw*qx"
  Divide2/1 -> Product1/1, Product2/2, Product5/2, Square1/1  "qy"
  Reshape/1 -> eulers_ZXY/1  "eulers_ZXY"
  Product1/1 -> Add/2  "qy*qz"
  Divide1/1 -> Product3/1, Product2/1, Product/2, Square2/1  "qx"
  Square6/1 -> Add5/1  "qw2"
  Asin/1 -> Vector Concatenate1/2  "Roll"
  Square5/1 -> Add5/2  "qx2"
  Asin1/1 -> Vector Concatenate1/1  "Yaw"
  Product4/1 -> Add2/2  "qw*qz"
  Multiport Selector/2 -> Square5/1, Divide1/1  "qx"
  Product2/1 -> Add2/1  "qx*qy"
  Product3/1 -> Add1/1  "qx*qz"
  Gain/1 -> Asin/1
  Divide/1 -> Product5/1, Product4/1, Product/1  "qw"
  Gain3/1 -> Asin2/1
  Gain4/1 -> Bias1/1
  Divide3/1 -> Product3/2, Product1/2, Square/1, Product4/2  "qz"
  Square/1 -> Add3/2  "qz2"
  Add1/1 -> Gain3/1
  Bias1/1 -> Asin2/2
  Add2/1 -> Gain1/1
  Add4/1 -> Gain4/1
  Asin2/1 -> Vector Concatenate1/3  "Pitch"
  Multiport Selector/3 -> Divide2/1, Square4/1  "qy"
  Square3/1 -> Add5/4  "qz2"
  Square2/1 -> Add3/1, Add4/1  "qx2"
  Square1/1 -> Add4/2  "qy2"
  Vector Concatenate1/1 -> Transpose/1
  Bias/1 -> Asin1/2
  Gain2/1 -> Bias/1
  Add3/1 -> Gain2/1
  Gain1/1 -> Asin1/1
  Transpose/1 -> Reshape/1
  Product5/1 -> Add1/2  "qw*qy"

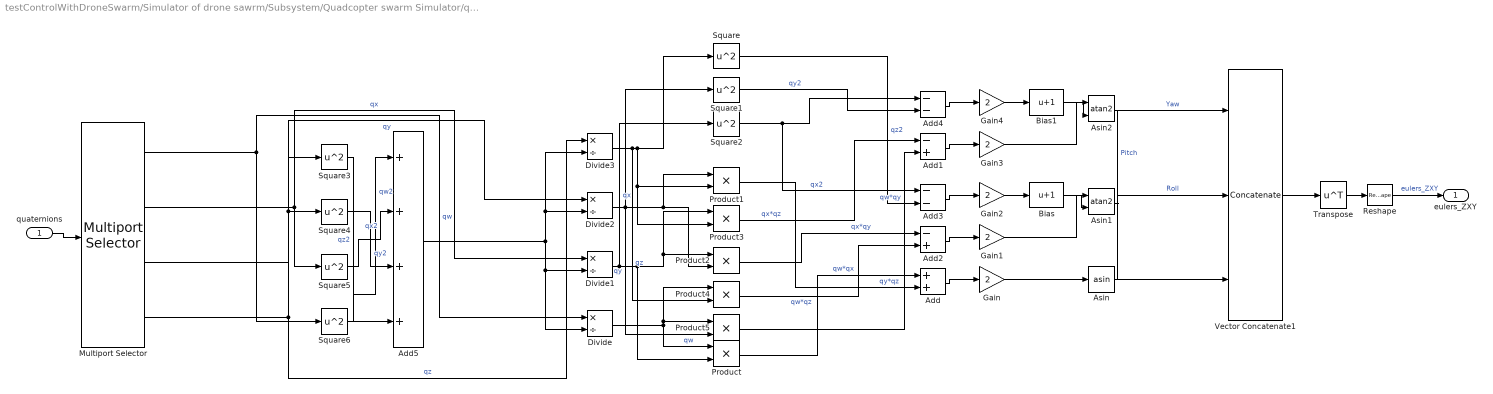
== system testControlWithDroneSwarm/Simulator of drone sawrm/Subsystem/Quadcopter swarm Simulator/quaternion2Euler1 ==
  quaternions : Inport
  Add : Sum
  Add1 : Sum  Inputs=-+
  Add2 : Sum  Inputs=-+
  Add3 : Sum  Inputs=--
  Add4 : Sum  Inputs=--
  Add5 : Sum  Inputs=++++
  Asin : Trigonometry  Operator=asin
  Asin1 : Trigonometry  Operator=atan2
  Asin2 : Trigonometry  Operator=atan2
  Bias : Bias  Bias=1
  Bias1 : Bias  Bias=1
  Divide{,1..3} (4 alike) : Product  Inputs=*/
  Gain{,1..4} (5 alike) : Gain  Gain=2
  Multiport Selector : dspindex/Multiport Selector  rowsOrCols=Rows  idxCellArray={ 1:4:4*number,2:4:4*number, 3:4:4*number, 4:4:4*number }  idxErrMode=Clip Index
  Product{,1..5} (6 alike) : Product
  Reshape : Reshape
  Square{,1..6} (7 alike) : Math  Operator=square  SaturateOnIntegerOverflow=on
  Transpose : Math  Operator=transpose  SaturateOnIntegerOverflow=on
  Vector Concatenate1 : Concatenate  NumInputs=3  Mode=Multidimensional array  ConcatenateDimension=2
  eulers_ZXY : Outport
  wires:
  Product5/1 -> Add1/2  "qw*qy"
  Transpose/1 -> Reshape/1
  Gain1/1 -> Asin1/1
  Add3/1 -> Gain2/1
  Gain2/1 -> Bias/1
  Bias/1 -> Asin1/2
  Vector Concatenate1/1 -> Transpose/1
  Square1/1 -> Add4/2  "qy2"
  Square2/1 -> Add4/1, Add3/1  "qx2"
  Square3/1 -> Add5/4  "qz2"
  Multiport Selector/3 -> Square4/1, Divide2/1  "qy"
  Asin2/1 -> Vector Concatenate1/3  "Pitch"
  Add4/1 -> Gain4/1
  Add2/1 -> Gain1/1
  Bias1/1 -> Asin2/2
  Add1/1 -> Gain3/1
  Square/1 -> Add3/2  "qz2"
  Divide3/1 -> Product4/2, Square/1, Product1/2, Product3/2  "qz"
  Gain4/1 -> Bias1/1
  Gain3/1 -> Asin2/1
  Divide/1 -> Product/1, Product4/1, Product5/1  "qw"
  Gain/1 -> Asin/1
  Product3/1 -> Add1/1  "qx*qz"
  Product2/1 -> Add2/1  "qx*qy"
  Multiport Selector/2 -> Divide1/1, Square5/1  "qx"
  Product4/1 -> Add2/2  "qw*qz"
  Asin1/1 -> Vector Concatenate1/1  "Yaw"
  Square5/1 -> Add5/2  "qx2"
  Asin/1 -> Vector Concatenate1/2  "Roll"
  Square6/1 -> Add5/1  "qw2"
  Divide1/1 -> Square2/1, Product/2, Product2/1, Product3/1  "qx"
  Product1/1 -> Add/2  "qy*qz"
  Reshape/1 -> eulers_ZXY/1  "eulers_ZXY"
  Divide2/1 -> Square1/1, Product5/2, Product2/2, Product1/1  "qy"
  Product/1 -> Add/1  "qw*qx"
  Multiport Selector/4 -> Square3/1, Divide3/1  "qz"
  quaternions/1 -> Multiport Selector/1
  Add/1 -> Gain/1
  Square4/1 -> Add5/3  "qy2"
  Add5/1 -> Divide2/2, Divide3/2, Divide/2, Divide1/2
  Multiport Selector/1 -> Square6/1, Divide/1  "qw"

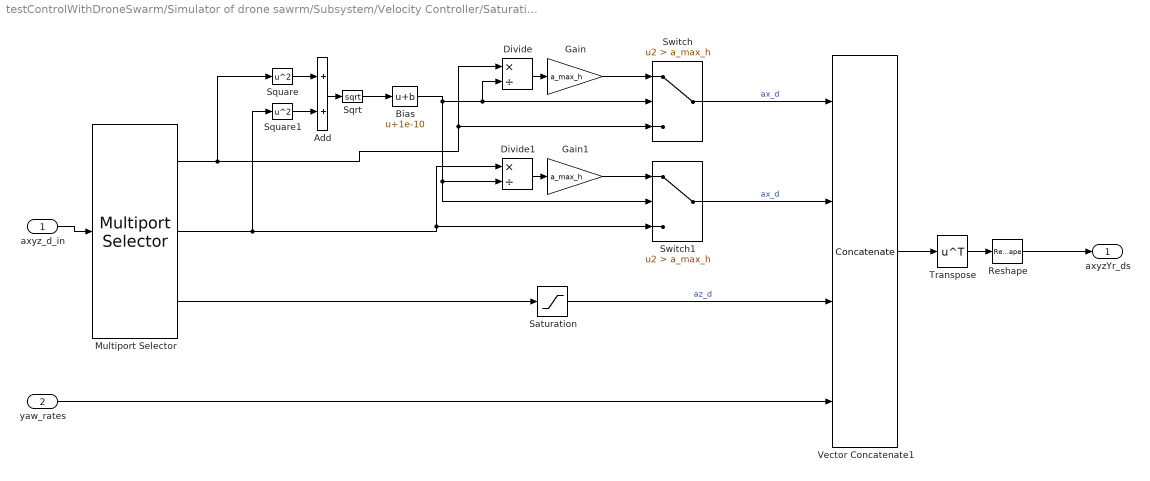
== system testControlWithDroneSwarm/Simulator of drone sawrm/Subsystem/Velocity Controller/Saturation_Acc ==
  axyz_d_in : Inport
  yaw_rates : Inport  Port=2
  Add : Sum
  Bias : Bias  Bias=1e-10
  Divide : Product  Inputs=*/
  Divide1 : Product  Inputs=*/
  Gain : Gain  Gain=a_max_h
  Gain1 : Gain  Gain=a_max_h
  Multiport Selector : dspindex/Multiport Selector  rowsOrCols=Rows  idxCellArray={ 1:3:3*number,2:3:3*number, 3:3:3*number}  idxErrMode=Clip Index
  Reshape : Reshape
  Saturation : Saturate  UpperLimit=a_max_v  LowerLimit=-a_max_v
  Sqrt : Sqrt  SaturateOnIntegerOverflow=on
  Square : Math  Operator=square  SaturateOnIntegerOverflow=on
  Square1 : Math  Operator=square  SaturateOnIntegerOverflow=on
  Switch : Switch  Criteria=u2 > Threshold  Threshold=a_max_h
  Switch1 : Switch  Criteria=u2 > Threshold  Threshold=a_max_h
  Transpose : Math  Operator=transpose  SaturateOnIntegerOverflow=on
  Vector Concatenate1 : Concatenate  NumInputs=4  Mode=Multidimensional array  ConcatenateDimension=2
  axyzYr_ds : Outport
  wires:
  Switch/1 -> Vector Concatenate1/1  "ax_d"
  Saturation/1 -> Vector Concatenate1/3  "az_d"
  Reshape/1 -> axyzYr_ds/1
  Multiport Selector/3 -> Saturation/1
  Gain/1 -> Switch/1
  Divide/1 -> Gain/1
  Multiport Selector/1 -> Switch/3, Divide/1, Square/1
  Add/1 -> Sqrt/1
  Square1/1 -> Add/2
  Square/1 -> Add/1
  axyz_d_in/1 -> Multiport Selector/1
  Sqrt/1 -> Bias/1
  Multiport Selector/2 -> Switch1/3, Divide1/1, Square1/1
  Divide1/1 -> Gain1/1
  Gain1/1 -> Switch1/1
  Switch1/1 -> Vector Concatenate1/2  "ax_d"
  Transpose/1 -> Reshape/1
  Vector Concatenate1/1 -> Transpose/1
  yaw_rates/1 -> Vector Concatenate1/4
  Bias/1 -> Switch/2, Divide/2, Switch1/2, Divide1/2

== matlab function testControlWithDroneSwarm/Simulator of drone sawrm/Subsystem/Commander/MATLAB Function ==
  settings: updateMethod=DISCRETE
  data: commands input; xyzYaw_ds output; states input; t input; vxyzYr_ds_fw output; axyz_ds_fw output
function [xyzYaw_ds, vxyzYr_ds_fw, axyz_ds_fw] = commander(commands, states,t)
persistent states_save  message_Ids_former t_start_Circle t_trigger v_save vx_save vy_save
number = size(states,2);
if isempty(states_save) || t < 0.1
    states_save = states;
    message_Ids_former = zeros(1,number)-1;
end
xyz_s = states(1:3,:);
% vxyz_s = states(4:6,:);
% axyz_s = states(7:9,:);
yrp_s = states(10:12,:);

xyzYaw_ds = [xyz_s;yrp_s(1,:)];
vxyzYr_ds_fw = zeros(4,number);
axyz_ds_fw   = zeros(3,number);



component_ids = commands(1,:);
message_ids = commands(2,:);
msgs = commands(3:6,:);

COMMAND_TYPE = 0;

Arming = 1;
Takeoff = 2;
Hover = 3;
Land = 4;
Position_control = 5;
Velocity_control = 6;
Velocity_horizontal_control = 7;
Acceleration_control = 8;

for id = 1:number
    component_id = component_ids(id);
    if component_id == COMMAND_TYPE
        message_id = message_ids(id);
        message_id_former = message_Ids_former(id);
        msg = msgs(:,id);
        switch message_id
            case Arming
                if message_id_former ~= message_id
                    fprintf("UAV %d armed.\n",int16(id));
                    states_save(:,id) = states(:,id);
                end
                xyzYaw_ds(:,id) = states_save([1,2,3,10],id);
            case Takeoff
                if message_id_former ~= message_id
%                     str = sprintf("UAV %d takeoff.",id);
%                     disp(str);
%                     disp(str);
                    fprintf("UAV %d takeoff.\n",int16(id));
                    states_save(:,id) = states(:,id);
                end
                xyzYaw_ds(:,id) = states_save([1,2,3,10],id);
                xyzYaw_ds(3,id) = msg(1);
            case Hover
                if message_id_former ~= message_id
%                     disp(['UAV ',num2str(id),' hover.']);
                    states_save(:,id) = states(:,id);
                end
                xyzYaw_ds(:,id) = states_save([1,2,3,10],id);
            case Land
                if message_id_former ~= message_id
%                     disp(['UAV ',num2str(id),' land.']);
                    states_save(:,id) = states(:,id);
                end
                xyzYaw_ds(:,id) = states_save([1,2,3,10],id);
                xyzYaw_ds(3,id) = msg(1);
            case Position_control
                if message_id_former ~= message_id
%                     disp(['UAV ',num2str(id),' position control.']);
                end
                xyzYaw_ds(:,id) = msg;
            case Velocity_control
                if message_id_former ~= message_id
%                     disp(['UAV ',num2str(id),' velocity control.']);
                end
                vxyzYr_ds_fw(:,id) = msg;
            case Velocity_horizontal_control
                if message_id_former ~= message_id
%                     disp(['UAV ',num2str(id),' velocity horizontal control.']);
                end
                vxyzYr_ds_fw([1,2,4],id) = msg([1,2,4]);
                xyzYaw_ds(3,id) = msg(3);
            case Acceleration_control
                if message_id_former ~= message_id
%                     disp(['UAV ',num2str(id),' acceleration control.']);
                end
                axyz_ds_fw(:,id) = msg(1:3);
        end
        message_Ids_former(id) = message_id;
    end
end

== matlab function testControlWithDroneSwarm/Commander/MATLAB Function ==
  data: message_id_s output; manual_id input; state_s input; msg_s output; map3d_faces input; map3d_struct input; t input; flag_alg input; dt input
function [message_id_s, msg_s] = swarm_algorithm(manual_id,state_s, map3d_faces, map3d_struct, t, flag_alg, dt)

number_all = size(state_s,2);
msg_s = zeros(4,number_all);
message_id_s = zeros(1,number_all);

% If the agent is not captured by mocap, its states are all 0. 
is_running = sum(abs(state_s(1:6,:)),1) > 0.001;

%%
% Value of rotary switch
manual_arming = 1;
manual_takeoff = 2;
manual_hover = 3;
manual_land = 4;
manual_alg = 5;
manual_test = 6;
% External control mode
Arming_type = 1;
Takeoff_type = 2;
Hover_type = 3;
Land_type = 4;
Position_control_type = 5;
Velocity_control_type = 6;
Velocity_horizontal_control_type = 7;

%
h_takeoff = 1.0;
h_land = 0.0;
switch manual_id
    case manual_arming
        message_id_s = Arming_type * ones(1,number_all);
        msg_s = zeros(4,number_all);
    case manual_takeoff
        message_id_s = Takeoff_type * ones(1,number_all);
        msg_s = zeros(4,number_all);
        msg_s(1,:) = h_takeoff;
    case manual_hover
        message_id_s = Hover_type * ones(1,number_all);
        msg_s = zeros(4,number_all);
    case manual_land
        message_id_s = Land_type * ones(1,number_all);
        msg_s = zeros(4,number_all);
        msg_s(1,:) = h_land;
    case manual_alg
        id_is_running = find(is_running);
%         vel_desired = zeros(2, length(id_is_running));
        
        if sensor_env_module_get_activate()
            motion_model_type = 0; %%%%%%%%%%%%%%%%%%%%
            sensor_data_s = sensor_env_module_get_data_all(state_s(:,id_is_running), motion_model_type, map3d_faces);
        else
            sensor_data_s = [];
        end
        [command_upper_s_isr,control_mode_s_u_isr] = ...
            swarm_module_generate_desire(t, state_s(:,id_is_running), flag_alg, dt, sensor_data_s);
        
        pos_desired_s_isr = command_upper_s_isr(1:4,:);
        vel_desired_s_isr = command_upper_s_isr(5:8,:);
  
        message_id_s(id_is_running) = control_mode_s_u_isr;
        control_mode_unique = unique(control_mode_s_u_isr);
        for c = 1:length(control_mode_unique)
            control_mode = control_mode_unique(c);
            id_selected_isr = find(control_mode_s_u_isr==control_mode);
            msg_s_isr = zeros(4,length(id_selected_isr));
            switch control_mode
                case Takeoff_type
                    message_id_s = Takeoff_type * ones(1,number_all);
                    msg_s_isr(1,:) = pos_desired_s_isr(3,id_selected_isr);
                case Land_type
                    message_id_s = Land_type * ones(1,number_all);
                    msg_s_isr(1,:) = pos_desired_s_isr(3,id_selected_isr);
                case Hover_type
                    message_id_s = Hover_type * ones(1,number_all);
                case Position_control_type
                    message_id_s = Land_type * ones(1,number_all);
                    msg_s_isr(:,:) = pos_desired_s_isr(:,id_selected_isr);
                case Velocity_control_type
                    message_id_s = Velocity_control_type * ones(1,number_all);
                    msg_s_isr(:,:) = vel_desired_s_isr(:,id_selected_isr);
                case Velocity_horizontal_control_type 
                    message_id_s = Velocity_horizontal_control_type * ones(1,number_all);
                    msg_s_isr([1,2,4],:) = vel_desired_s_isr([1,2,4],id_selected_isr);
                    msg_s_isr(3,:) = pos_desired_s_isr(3,id_selected_isr);
            end
            id_selected = id_is_running(id_selected_isr);
            msg_s(:,id_selected) = msg_s_isr;
        end
    case manual_test
        xyz_s = state_s(1:3,:);
        vxyz_s = state_s(4:6,:);
        id_is_running = find(is_running);
        num_is_runnning = length(id_is_running);
        xyz_s_is_running = xyz_s(:,is_running);
        vxyz_s_is_running = vxyz_s(:,is_running);
        velDesired = zeros(3,num_is_runnning);
        % Params
        v_flock = 0.4;
        z_d = 0.7;
        r_rep = 1.0;
        p_rep = 1.0;
        v_wall_0 = 0.4;
        x_range_wall = [-1.5,1.5];
        y_range_wall = [-1.5,1.5];
        v_max = 0.4;
        % =============Behaviors=============
        % Alignment
        v_vist = mean(vxyz_s_is_running(1:2,:),2);
        v_vist_norm = norm(v_vist);
        if v_vist_norm>0
            v_vist = v_vist/v_vist_norm * v_flock;
        else
            v_vist = rand(2,1);
            v_vist = v_vist/norm(v_vist) * v_flock;
        end
        % Repulsion
        v_rep = zeros(2,num_is_runnning);
        x_ij = repmat(xyz_s_is_running(1,:),num_is_runnning,1) -...
            repmat(xyz_s_is_running(1,:)',1,num_is_runnning);
        y_ij = repmat(xyz_s_is_running(2,:),num_is_runnning,1) -...
            repmat(xyz_s_is_running(2,:)',1,num_is_runnning);
        d_ij = sqrt(x_ij.^2 + y_ij.^2);
        d_ij(1:num_is_runnning+1:num_is_runnning^2) = r_rep*100;
        in_rep = double(d_ij < r_rep);
        v_rep(1,:) = p_rep*sum( (r_rep - d_ij).*x_ij./d_ij.*in_rep ,1);
        v_rep(2,:) = p_rep*sum( (r_rep - d_ij).*y_ij./d_ij.*in_rep ,1);
        % Wall avoidance
        v_wall = zeros(2,num_is_runnning);
        v_wall(1,:) = double(xyz_s_is_running(1,:) < x_range_wall(1)) * 1.0 + ...
            double(xyz_s_is_running(1,:) > x_range_wall(2)) * (-1.0);
        v_wall(2,:) = double(xyz_s_is_running(2,:) < y_range_wall(1)) * 1.0 + ...
            double(xyz_s_is_running(2,:) > y_range_wall(2)) * (-1.0);
        v_wall_norm = sqrt(sum(v_wall.^2,1));
        v_wall_norm(v_wall_norm==0) = 10;
        v_wall = v_wall_0*v_wall./v_wall_norm;

        % Combination
        velDesired(1:2,:) = repmat(v_vist,1,num_is_runnning) + v_rep + v_wall;
        velDesired_norm = sqrt(sum(velDesired(1:2,:).^2,1));
        temp = find(velDesired_norm>v_max);
        if ~isempty(temp)
            velDesired(1:2,temp) = v_max*velDesired(1:2,temp)./velDesired_norm(temp);
        end
        %
%         message_id_s(id_is_running) = Velocity_horizontal_control_type;
%         msg_s(1,id_is_running) = velDesired(1,:);
%         msg_s(2,id_is_running) = velDesired(2,:);
%         msg_s(3,id_is_running) = z_d; % z_d
%         msg_s(4,id_is_running) = 0.0; % yaw_rate_d
        %
        message_id_s(id_is_running) = Velocity_control_type;
        msg_s(1,id_is_running) = velDesired(1,:);
        msg_s(2,id_is_running) = velDesired(2,:);
        msg_s(3,id_is_running) = 0.1*sin(t); % vz_d
        msg_s(4,id_is_running) = 0.0; % yaw_rate_d
    otherwise

end

== matlab function testControlWithDroneSwarm/Simulator of drone sawrm/Subsystem/Display/MATLAB Function ==
  settings: updateMethod=DISCRETE
  data: states input; lenArm input; t input
function fcn(states,lenArm, t)
persistent t_last count
figure(1)
if isempty(t_last)
    t_last = 0;
    count = 1;
    myFigure = figure(1);
    cla(myFigure);
    hold on
    grid on
    box on
    axis equal
    view([-35,35]);
    xlim([-4,4]);
    ylim([-4,4]);
    zlim([0,3]);
    xlabel('X Position (m)')
    ylabel('Y Position (m)')
    plotMultiQuadcopters(myFigure,states,lenArm);
end
if t - t_last > 0.5
    myFigure = figure(1);
    cla(myFigure);
    plotMultiQuadcopters(myFigure,states,lenArm);
%     xlim([-2,2]);
%     ylim([-3.5,3]);
%     zlim([0,2]);
    t_last = t;
end
count = count + 1;

== matlab function testControlWithDroneSwarm/Map update/MATLAB Function ==
  data: t input; map3d_faces output; sample_time_control input; map3d_faces_0 input; map3d_struct_0 input; map3d_struct output
function [map3d_faces,map3d_struct] = fcn(t, sample_time_control,map3d_faces_0, map3d_struct_0)

persistent map3d_faces_new map3d_struct_new
if isempty(map3d_faces_new) || t==0
    map3d_faces_new = map3d_faces_0;
    map3d_struct_new = map3d_struct_0;
end


[map3d_faces_new,map3d_struct_new] = map_module_update_map3d(t, sample_time_control,map3d_faces_new, map3d_struct_new);

map3d_faces = map3d_faces_new;
map3d_struct = map3d_struct_new;

== matlab function testControlWithDroneSwarm/Visualization/MATLAB Function ==
  data: t input; dt input; states input; map3d_faces input; map3d_struct input
function fcn(t, dt, states, map3d_faces, map3d_struct)
coder.extrinsic('draw_environment');
coder.extrinsic('adjust_figure_axis');
coder.extrinsic('num2str');
coder.extrinsic('draw_body');

persistent f_1 a_1

[activate_plot,...
    time_interval_plot,...
    activate_trajectory,...
    follow_agent,...
    activate_save_figure,...
    activate_save_video,...
    dim_visual,...
    time_interval_trajectory,...
    video_speed] = visual_module_parameters();

if ~activate_plot
    return
end

if t == 0 || isempty(f_1) || isempty(a_1)
    start_and_end = 1;
    f_1 = figure;
    a_1 = gca;
    hold(a_1,'on'); grid(a_1,'on'); box(a_1,'on')
    axis(a_1,'equal')
    xlabel(a_1,'X Position (m)');
    ylabel(a_1,'Y Position (m)');
    if dim_visual == 3
        zlabel(a_1,'Z Position (m)');
        view(a_1,[-45,30]);
    end
    title(a_1,['Elapsed time ',num2str(t,"%.2f"),' s'])
    [x_range,y_range,z_range] = get_range(states, map3d_faces);
    xlim(a_1,x_range);
    ylim(a_1,y_range);
    zlim(a_1,z_range);
else
    start_and_end = 0;
end

flag_motion_model = 1;
if visual_module_get_activate(dt,t,start_and_end)
    draw_environment(a_1, map3d_faces, map3d_struct, [], dim_visual);

    num = size(states,2);
    len_arm = 0.1;
    color_s_bodies = zeros(3,num);
    draw_body(a_1, states, dim_visual, flag_motion_model, len_arm, color_s_bodies);
    title(a_1,['Elapsed time ',num2str(t,"%.2f"),' s'])
    [x_range,y_range,z_range] = get_range(states, map3d_faces);
    xlim(a_1,x_range);
    ylim(a_1,y_range);
    zlim(a_1,z_range);
end

    function [x_range,y_range,z_range] = get_range(states, map3d_faces)
        if ~isempty(map3d_faces)
            x_range = [min(map3d_faces(1:3:9,:),[],'all'),max(map3d_faces(1:3:9,:),[],'all')];
            y_range = [min(map3d_faces(2:3:9,:),[],'all'),max(map3d_faces(2:3:9,:),[],'all')];
            z_range = [min(map3d_faces(3:3:9,:),[],'all'),max(map3d_faces(3:3:9,:),[],'all')];
        else
            x_range = [min(states(1,:)),max(states(1,:))];
            y_range = [min(states(2,:)),max(states(2,:))];
            z_range = [min(states(3,:)),max(states(3,:))];
        end
        if x_range(2) - x_range(1) <=0
            x_range = [0,1];
        end
        if y_range(2) - y_range(1) <=0
            y_range = [0,1];
        end
        if z_range(2) - z_range(1) <=0
            z_range = [0,1];
        end
    end
end
